simulink model "test_10gbe_mux_pack"  (Simulink 6.2)
settings: Solver=ode45  StartTime=0.0  StopTime=24000  RelTol=1e-3
libraries: xbsIndex_r3 x358, xps_library x31, casper_library x9
(part 1 of 3)
settings Model: LastModifiedBy=manley
settings DebuggingCC: SolverPrmCheckMsg=warning

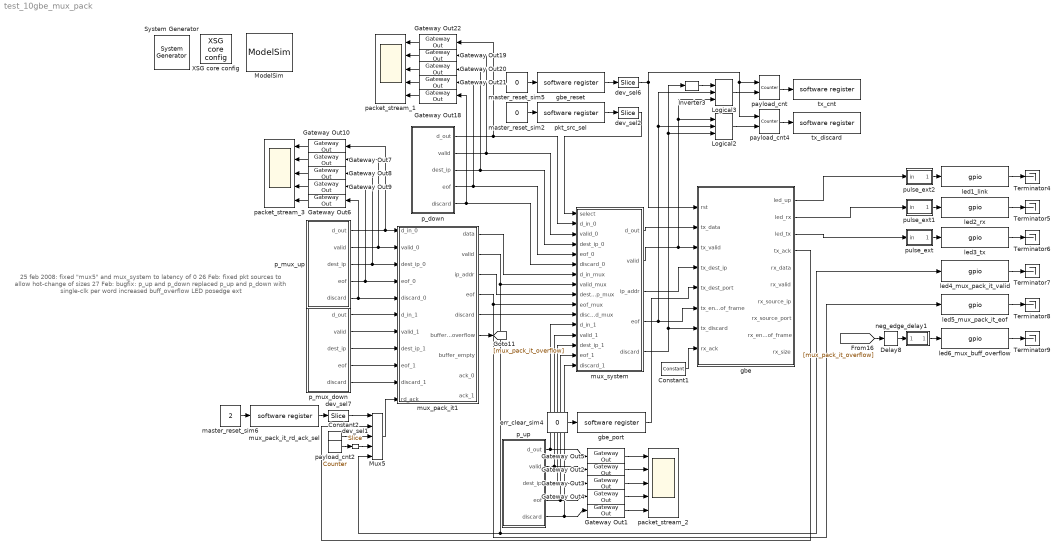
== system test_10gbe_mux_pack ==
  note: 25 feb 2008:
      | fixed "mux5" and mux_system to latency of 0
      |
      | 26 Feb:
      | fixed pkt sources to allow hot-change of sizes
      |
      | 27 Feb:
      | bugfix: p_up and p_down
      | replaced p_up and p_down with single-clk per word
      | increased buff_overflow LED posedge ext
  " System Generator" : xbsIndex_r3/ System Generator  Tag=genX  xilinxfamily=Virtex2P  part=xc2vp70  speed=-7  package=ff1704  synthesis_tool=XST  directory=./test_10gbe_mux_pack/sysgen  testbench=off  simulink_period=1  sysclk_period=4.878  incr_netlist=off  trim_vbits=Everywhere in SubSystem  dbl_ovrd=According to Block Masks  core_generation=According to Block Masks  run_coregen=off  deprecated_control=off  eval_field=0
      settings: AttributesFormatString=System\nGenerator
  Constant1 : xbsIndex_r3/Constant  const=1  equ=P=C  arith_type=Boolean  n_bits=1  bin_pt=0  opselect=C  inp2=PCIN>>17  opr=+  inp1=P  carry=CIN  iostate=0  explicit_period=on  period=1  dbl_ovrd=off
  Constant2 : xbsIndex_r3/Constant  const=1  equ=P=C  arith_type=Boolean  n_bits=1  bin_pt=0  opselect=C  inp2=PCIN>>17  opr=+  inp1=P  carry=CIN  iostate=0  explicit_period=on  period=1  dbl_ovrd=off
  Delay8 : xbsIndex_r3/Delay  latency=1  reg_retiming=off  explicit_period=off  period=1  en=off  accept_only_valid=off  init_zero=on  dbl_ovrd=off  show_param=off
      settings: xl_area=[0, 0, 0, 0, 0, 0, 0]
  Gateway Out{1..5} (5 alike) : xbsIndex_r3/Gateway Out  output_type=Double  nbits=8  bin_pt=6  arith_type=Boolean  quantization=Truncate  overflow=Wrap  hdl_port=on  timing_constraint=None  locs_specified=off  LOCs={}  needs_fixed_name=off  show_param=off
      settings: xl_area=[0, 0, 0, 0, 0, 0, 0]
  Gateway Out{6..10,18..22} (10 alike) : xbsIndex_r3/Gateway Out  Orientation=left  output_type=Double  nbits=8  bin_pt=6  arith_type=Boolean  quantization=Truncate  overflow=Wrap  hdl_port=on  timing_constraint=None  locs_specified=off  LOCs={}  needs_fixed_name=off  show_param=off
      settings: xl_area=[0, 0, 0, 0, 0, 0, 0]
  Inverter3 : xbsIndex_r3/Inverter  latency=0  explicit_period=off  period=1  en=off  dbl_ovrd=off  show_param=off
      settings: xl_area=[0, 0, 0, 0, 0, 0, 0]
  Logical2 : xbsIndex_r3/Logical  logical_function=AND  inputs=3  precision=Full  arith_type=Unsigned  n_bits=8  bin_pt=2  align_bp=on  latency=0  explicit_period=on  period=1  en=off  dbl_ovrd=off  show_param=off
      settings: xl_area=[0, 0, 0, 0, 0, 0, 0]
  Logical3 : xbsIndex_r3/Logical  logical_function=AND  inputs=3  precision=Full  arith_type=Unsigned  n_bits=8  bin_pt=2  align_bp=on  latency=0  explicit_period=on  period=1  en=off  dbl_ovrd=off  show_param=off
      settings: xl_area=[0, 0, 0, 0, 0, 0, 0]
  ModelSim : xbsIndex_r3/ModelSim  dir=./modelsim  waveform=on  leave_open=on  skip_compile=off  custom_scripts=off  startup_timeout=40
  Mux5 : xbsIndex_r3/Mux  inputs=4  precision=Full  arith_type="Signed  (2's comp)"  n_bits=8  bin_pt=2  quantization=Truncate  overflow=Wrap  latency=0  explicit_period=on  period=1  en=off  dbl_ovrd=off  show_param=off  mux_type=off  use_rpm=off  gen_core=off
      settings: xl_area=[0, 0, 0, 0, 0, 0, 0]
  Terminator{4..9} (6 alike) : Terminator
  XSG core config : xps_library/XSG core config  Tag=xps:xsg  hw_sys=BEE2_usr  ibob_linux=off  clk_src=sys_clk2x  gpio_clk_io_group=iBOB:sma  gpio_clk_bit_index=0  clk_rate=205  sample_period=1  synthesis_tool=XST  mpc_type=powerpc405
  dev_sel1 : xbsIndex_r3/Slice  mode=Lower Bit Location + Width  nbits=1  bit1=0  base1=MSB of Input  bit0=0  base0=LSB of Input  boolean_output=on  explicit_period=off  period=1  dbl_ovrd=off
  dev_sel2 : xbsIndex_r3/Slice  mode=Lower Bit Location + Width  nbits=2  bit1=0  base1=MSB of Input  bit0=0  base0=LSB of Input  boolean_output=off  explicit_period=off  period=1  dbl_ovrd=off
  dev_sel6 : xbsIndex_r3/Slice  mode=Lower Bit Location + Width  nbits=1  bit1=0  base1=MSB of Input  bit0=0  base0=LSB of Input  boolean_output=on  explicit_period=off  period=1  dbl_ovrd=off
  dev_sel7 : xbsIndex_r3/Slice  mode=Lower Bit Location + Width  nbits=2  bit1=0  base1=MSB of Input  bit0=0  base0=LSB of Input  boolean_output=off  explicit_period=off  period=1  dbl_ovrd=off
  err_clear_sim4 : Constant  Value=0
  gbe : Subsystem  Tag=xps:tengbe  AncestorBlock=xps_library/ten_GbE  mask{port=BEE2_usr:2, mac_lite=on, show_param=off, pre_emph=3, swing=800}
      mask prompts: mac_lite "Use light-weight MAC: Warning --> it DOES NOT check any CRC on receive"; show_param "---------------------- Show Implementation Parameters -----------------------------------------------------------------------------------"; pre_emph "Pre-emphasis"; swing "Differential swing"
      mask init:
      | tengbe_mask;
      mask StyleString: popup(iBOB:0|iBOB:1|BEE2_ctrl:0|BEE2_ctrl:1|BEE2_usr:0|BEE2_usr:1|BEE2_usr:2|BEE2_usr:3|CORR:0),checkbox,checkbox,popup(0|1|2|3),popup(400|500|600|700|800)
      mask CallbackString:
      | ||myname=gcb;
      | if strcmp(get_param(myname, 'show_param'), 'on')
      |     set_param(myname, 'MaskVisibilities', {'on','on','on','on', 'on'});
      | else
      |     set_param(myname, 'MaskVisibilities', {'on','on','on','off','off'});
      | end||
  gbe_port : xps_library/software register  Tag=xps:sw_reg  io_dir=From Processor  arith_type=Unsigned  bitwidth=32  bin_pt=0  sample_period=1  gw_name=test_10gbe_mux_pack_gbe_port_user_data_out
  gbe_reset : xps_library/software register  Tag=xps:sw_reg  io_dir=From Processor  arith_type=Unsigned  bitwidth=32  bin_pt=0  sample_period=1  gw_name=test_10gbe_mux_pack_gbe_reset_user_data_out
  led1_link : xps_library/gpio  Tag=xps:gpio  io_group=BEE2_usr:led  io_dir=out  arith_type=Boolean  bitwidth=1  bin_pt=0  bit_index=0  sample_period=1  use_single_ended=off  use_ddr=off  reg_iob=off  reg_clk_phase=0  termination=None
  led2_rx : xps_library/gpio  Tag=xps:gpio  io_group=BEE2_usr:led  io_dir=out  arith_type=Boolean  bitwidth=1  bin_pt=0  bit_index=1  sample_period=1  use_single_ended=off  use_ddr=off  reg_iob=off  reg_clk_phase=0  termination=None
  led3_tx : xps_library/gpio  Tag=xps:gpio  io_group=BEE2_usr:led  io_dir=out  arith_type=Boolean  bitwidth=1  bin_pt=0  bit_index=2  sample_period=1  use_single_ended=off  use_ddr=off  reg_iob=off  reg_clk_phase=0  termination=None
  led4_mux_pack_it_valid : xps_library/gpio  Tag=xps:gpio  io_group=BEE2_usr:led  io_dir=out  arith_type=Boolean  bitwidth=1  bin_pt=0  bit_index=3  sample_period=1  use_single_ended=off  use_ddr=off  reg_iob=off  reg_clk_phase=0  termination=None
  led5_mux_pack_it_eof : xps_library/gpio  Tag=xps:gpio  io_group=BEE2_usr:led  io_dir=out  arith_type=Boolean  bitwidth=1  bin_pt=0  bit_index=4  sample_period=1  use_single_ended=off  use_ddr=off  reg_iob=off  reg_clk_phase=0  termination=None
  led6_mux_buff_overflow : xps_library/gpio  Tag=xps:gpio  io_group=BEE2_usr:led  io_dir=out  arith_type=Boolean  bitwidth=1  bin_pt=0  bit_index=5  sample_period=1  use_single_ended=off  use_ddr=off  reg_iob=off  reg_clk_phase=0  termination=None
  master_reset_sim2 : Constant  Value=0
  master_reset_sim5 : Constant  Value=0
  master_reset_sim6 : Constant  Value=2
  mux_pack_it1 : Subsystem  mask(mux_packets){max_packet_size_0=1500, min_packet_size_0=50, max_packet_size_1=1500, min_packet_size_1=50}
      mask prompts: max_packet_size_0 "Input 0: Maximum single packet size (words)"; min_packet_size_0 "Input 0: Minimum single packet size (words)"; max_packet_size_1 "Input 1: Maximum single packet size (words)"; min_packet_size_1 "Input 1: Minimum single packet size (words)"
      mask help: This block allows you to mux together two data streams to be sent to the 10GbE core
  mux_pack_it_rd_ack_sel : xps_library/software register  Tag=xps:sw_reg  io_dir=From Processor  arith_type=Unsigned  bitwidth=32  bin_pt=0  sample_period=1  gw_name=test_10gbe_mux_pack_mux_pack_it_rd_ack_sel_user_data_out
  mux_system : Subsystem
  neg_edge_delay1 : Subsystem  AncestorBlock=casper_library/Misc/pulse_ext  mask(pulse_ext){pulse_len=2^27}
      mask prompts: pulse_len "Length of Pulse"
      mask help:
      | Extends a boolean signal to be high for the specified number of clocks after
      | the last high input.
      mask init:
      | bits = ceil(log2(pulse_len+1));
      mask Help: eval('xlWeb([getenv(''MLIB_ROOT''), ''\casper_library\doc\pulse_ext_usage.html''])')
  p_down : Subsystem
  p_mux_down : Subsystem
  p_mux_up : Subsystem
  p_up : Subsystem
  packet_stream_1 : Scope  NumInputPorts=5
      settings: YMin=4490~0~3.35544e+008~0~-1  YMax=4600~1~3.35544e+008~1~1
  packet_stream_2 : Scope  NumInputPorts=5
      settings: YMin=600~0~3.35544e+008~0~-1  YMax=710~1~3.35544e+008~1~1
  packet_stream_3 : Scope  NumInputPorts=5
      settings: YMin=800~0~3.18767e+008~0~-1  YMax=910~1~3.52321e+008~1~1  SaveName=ScopeData2
  payload_cnt : xbsIndex_r3/Counter  cnt_type=Free Running  n_bits=32  bin_pt=0  arith_type=Unsigned  start_count=0  cnt_to=0  cnt_by_val=1  operation=Up  explicit_period=off  period=1  load_pin=off  rst=on  en=on  dbl_ovrd=off  show_param=off  use_rpm=on  gen_core=off
      settings: xl_area=[0, 0, 0, 0, 0, 0, 0]
  payload_cnt2 : xbsIndex_r3/Counter  cnt_type=Free Running  n_bits=2  bin_pt=0  arith_type=Unsigned  start_count=0  cnt_to=0  cnt_by_val=1  operation=Up  explicit_period=off  period=1  load_pin=off  rst=off  en=off  dbl_ovrd=off  show_param=off  use_rpm=on  gen_core=off
      settings: xl_area=[0, 0, 0, 0, 0, 0, 0]
  payload_cnt4 : xbsIndex_r3/Counter  cnt_type=Free Running  n_bits=32  bin_pt=0  arith_type=Unsigned  start_count=0  cnt_to=0  cnt_by_val=1  operation=Up  explicit_period=off  period=1  load_pin=off  rst=on  en=on  dbl_ovrd=off  show_param=off  use_rpm=on  gen_core=off
      settings: xl_area=[0, 0, 0, 0, 0, 0, 0]
  pkt_src_sel : xps_library/software register  Tag=xps:sw_reg  io_dir=From Processor  arith_type=Unsigned  bitwidth=32  bin_pt=0  sample_period=1  gw_name=test_10gbe_mux_pack_pkt_src_sel_user_data_out
  pulse_ext : Subsystem  mask{pulse_len=2^23}
      mask prompts: pulse_len "Length of Pulse"
      mask init:
      | bits = ceil(log2(pulse_len));
  pulse_ext1 : Subsystem  mask{pulse_len=2^23}
      mask prompts: pulse_len "Length of Pulse"
      mask init:
      | bits = ceil(log2(pulse_len));
  pulse_ext2 : Subsystem  mask{pulse_len=2^23}
      mask prompts: pulse_len "Length of Pulse"
      mask init:
      | bits = ceil(log2(pulse_len));
  tx_cnt : xps_library/software register  Tag=xps:sw_reg  io_dir=To Processor  arith_type=Unsigned  bitwidth=32  bin_pt=0  sample_period=1  gw_name=test_10gbe_mux_pack_tx_cnt_user_data_in
  tx_discard : xps_library/software register  Tag=xps:sw_reg  io_dir=To Processor  arith_type=Unsigned  bitwidth=32  bin_pt=0  sample_period=1  gw_name=test_10gbe_mux_pack_tx_discard_user_data_in
  wires:
  p_down/1(d_out) -> Gateway Out22/1, mux_system/2(d_in_0)
  p_down/2(valid) -> Gateway Out19/1, mux_system/3(valid_0)
  p_down/3(dest_ip) -> Gateway Out20/1, mux_system/4(dest_ip_0)
  p_down/4(eof) -> Gateway Out21/1, mux_system/5(eof_0)
  p_down/5(discard) -> Gateway Out18/1, mux_system/6(discard_0)
  p_up/1(d_out) -> Gateway Out5/1, mux_system/12(d_in_1)
  p_up/2(valid) -> Gateway Out2/1, mux_system/13(valid_1)
  p_up/3(dest_ip) -> Gateway Out3/1, mux_system/14(dest_ip_1)
  p_up/4(eof) -> Gateway Out4/1, mux_system/15(eof_1)
  p_up/5(discard) -> Gateway Out1/1, mux_system/16(discard_1)
  dev_sel6/1 -> gbe/1(rst), payload_cnt/1, payload_cnt4/1
  mux_system/1(d_out) -> gbe/2(tx_data)
  mux_system/2(valid) -> gbe/3(tx_valid), Logical2/1, Logical3/3
  mux_pack_it1/6(buffer_overflow) -> [mux_pack_it_overflow]
  mux_system/3(ip_addr) -> gbe/4(tx_dest_ip)
  mux_system/4(eof) -> Logical2/2, Logical3/2, gbe/6(tx_end_of_frame)
  mux_system/5(discard) -> Inverter3/1, Logical2/3, gbe/7(tx_discard)
  mux_pack_it1/1(data) -> mux_system/7(d_in_mux)
  mux_pack_it1/2(valid) -> Mux5/5, led4_mux_pack_it_valid/1, mux_system/8(valid_mux)
  mux_pack_it1/3(ip_addr) -> mux_system/9(dest_ip_mux)
  mux_pack_it1/4(eof) -> led5_mux_pack_it_eof/1, mux_system/10(eof_mux)
  mux_pack_it1/5(discard) -> mux_system/11(discard_mux)
  Inverter3/1 -> Logical3/1
  payload_cnt/1 -> tx_cnt/1
  payload_cnt4/1 -> tx_discard/1
  Logical2/1 -> payload_cnt4/2
  Logical3/1 -> payload_cnt/2
  master_reset_sim2/1 -> pkt_src_sel/1
  pkt_src_sel/1 -> dev_sel2/1
  master_reset_sim5/1 -> gbe_reset/1
  gbe_reset/1 -> dev_sel6/1
  pulse_ext/1(out) -> led3_tx/1
  pulse_ext1/1(out) -> led2_rx/1
  pulse_ext2/1(out) -> led1_link/1
  led1_link/1 -> Terminator4/1
  led2_rx/1 -> Terminator5/1
  led3_tx/1 -> Terminator6/1
  led4_mux_pack_it_valid/1 -> Terminator7/1
  led5_mux_pack_it_eof/1 -> Terminator8/1
  led6_mux_buff_overflow/1 -> Terminator9/1
  Delay8/1 -> neg_edge_delay1/1(in)
  neg_edge_delay1/1(out) -> led6_mux_buff_overflow/1
  gbe/1(led_up) -> pulse_ext2/1(in)
  gbe/2(led_rx) -> pulse_ext1/1(in)
  gbe/3(led_tx) -> pulse_ext/1(in)
  Constant1/1 -> gbe/8(rx_ack)
  err_clear_sim4/1 -> gbe_port/1
  gbe_port/1 -> gbe/5(tx_dest_port)
  [mux_pack_it_overflow] -> Delay8/1
  master_reset_sim6/1 -> mux_pack_it_rd_ack_sel/1
  mux_pack_it_rd_ack_sel/1 -> dev_sel7/1
  dev_sel7/1 -> Mux5/1
  Constant2/1 -> Mux5/3
  Mux5/1 -> mux_pack_it1/11(rd_ack)
  dev_sel2/1 -> mux_system/1(select)
  Gateway Out22/1 -> packet_stream_1/1
  Gateway Out19/1 -> packet_stream_1/2
  Gateway Out20/1 -> packet_stream_1/3
  Gateway Out21/1 -> packet_stream_1/4
  Gateway Out18/1 -> packet_stream_1/5
  Gateway Out5/1 -> packet_stream_2/1
  Gateway Out2/1 -> packet_stream_2/2
  Gateway Out3/1 -> packet_stream_2/3
  Gateway Out4/1 -> packet_stream_2/4
  Gateway Out1/1 -> packet_stream_2/5
  gbe/4(tx_ack) -> Mux5/2
  payload_cnt2/1 -> dev_sel1/1
  dev_sel1/1 -> Mux5/4
  p_mux_up/1(d_out) -> mux_pack_it1/1(d_in_0), Gateway Out10/1
  p_mux_up/2(valid) -> mux_pack_it1/2(valid_0), Gateway Out7/1
  p_mux_up/3(dest_ip) -> mux_pack_it1/3(dest_ip_0), Gateway Out8/1
  p_mux_up/4(eof) -> mux_pack_it1/4(eof_0), Gateway Out9/1
  p_mux_up/5(discard) -> mux_pack_it1/5(discard_0), Gateway Out6/1
  p_mux_down/1(d_out) -> mux_pack_it1/6(d_in_1)
  p_mux_down/2(valid) -> mux_pack_it1/7(valid_1)
  p_mux_down/3(dest_ip) -> mux_pack_it1/8(dest_ip_1)
  p_mux_down/4(eof) -> mux_pack_it1/9(eof_1)
  p_mux_down/5(discard) -> mux_pack_it1/10(discard_1)
  Gateway Out10/1 -> packet_stream_3/1
  Gateway Out7/1 -> packet_stream_3/2
  Gateway Out8/1 -> packet_stream_3/3
  Gateway Out9/1 -> packet_stream_3/4
  Gateway Out6/1 -> packet_stream_3/5

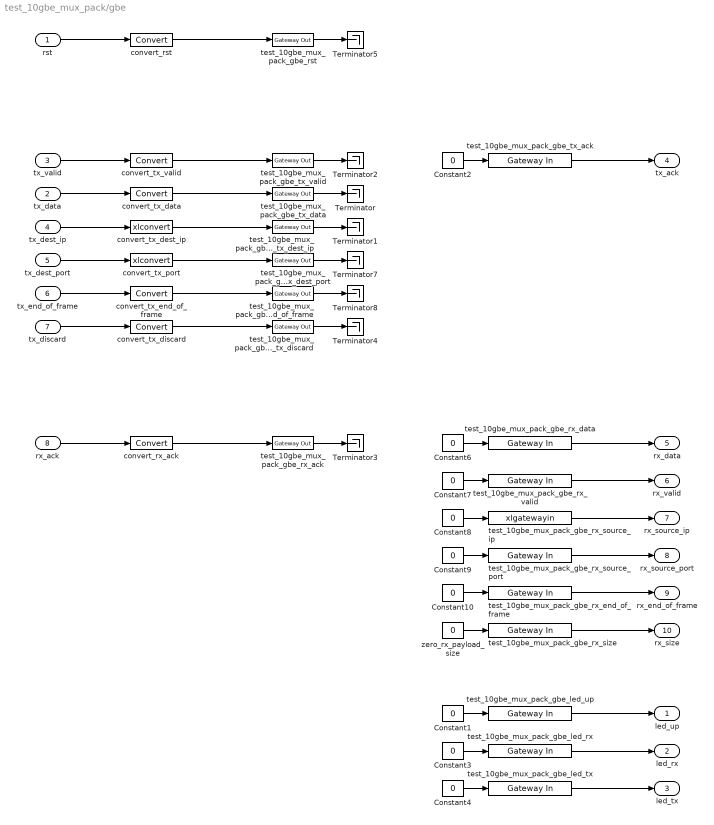
== system test_10gbe_mux_pack/gbe ==
  rst : Inport  Port=1  LatchInput=off
  tx_data : Inport  Port=2  LatchInput=off
  tx_valid : Inport  Port=3  LatchInput=off
  tx_dest_ip : Inport  Port=4  LatchInput=off
  tx_dest_port : Inport  Port=5  LatchInput=off
  tx_end_of_frame : Inport  Port=6  LatchInput=off
  tx_discard : Inport  Port=7  LatchInput=off
  rx_ack : Inport  Port=8  LatchInput=off
  Constant{1..4,6..10} (9 alike) : Constant  Value=0
  Terminator{,1..5,7..8} (8 alike) : Terminator
  convert_rst : xbsIndex_r3/Convert  arith_type=Boolean  n_bits=64  bin_pt=0  quantization=Truncate  overflow=Wrap  latency=0  explicit_period=off  period=1  dbl_ovrd=off  show_param=off  inserted_by_tool=off  pipeline=off
      settings: xl_area=[0, 0, 0, 0, 0, 0, 0]
  convert_rx_ack : xbsIndex_r3/Convert  arith_type=Boolean  n_bits=64  bin_pt=0  quantization=Truncate  overflow=Wrap  latency=0  explicit_period=off  period=1  dbl_ovrd=off  show_param=off  inserted_by_tool=off  pipeline=off
      settings: xl_area=[0, 0, 0, 0, 0, 0, 0]
  convert_tx_data : xbsIndex_r3/Convert  arith_type=Unsigned  n_bits=64  bin_pt=0  quantization=Truncate  overflow=Wrap  latency=0  explicit_period=off  period=1  dbl_ovrd=off  show_param=off  inserted_by_tool=off  pipeline=off
      settings: xl_area=[0, 0, 0, 0, 0, 0, 0]
  convert_tx_dest_ip : S-Function  AncestorBlock=xbsIndex_r3/Convert  FunctionName=xlconvert  Parameters=sfcn_mwsv__  mask(Xilinx Converter Block){arith_type=Unsigned, n_bits=32, bin_pt=0, quantization=Truncate, overflow=Wrap, latency=0, explicit_period=off, period=1, dbl_ovrd=off, show_param=off, inserted_by_tool=off, pipeline=off, xl_area=[0, 0, 0, 0, 0, 0, 0], xl_use_area=off}
      mask prompts: arith_type "Output Type"; n_bits "Number of Bits"; bin_pt "Binary Point"; quantization "Quantization Behavior"; overflow "Overflow Behavior"; explicit_period "Use Explicit Sample Period"; period "Sample Period"; dbl_ovrd "Override with Doubles"; show_param "---------------------- Show Implementation Parameters -----------------------------------------------------------------------------------"; inserted_by_tool "Hidden Parameter:  inserted_by_tool"; pipeline "Pipeline to Greatest Extent Possible"; xl_area "FPGA Area [Slices, FFs, BRAMs, LUTs, IOBs, Emb. Mults, TBUFs]"; xl_use_area "Use Area Above For Estimation"
      mask help:
      | Type conversion block. The input is presented at the output after quantization and overflow effects.
      |
      | Hardware notes: Additional hardware is used when rounding or saturation is selected and output width is less than the input width.
      mask init:
      | [designRoot, family, part, speed, package, simulinkPeriod, sysclkPeriod, dbl_ovrd, trimVbit] = xlSysgenSettings(gcb,1,1);
      | if (arith_type==1)
      |   bool = 1;
      | else
      |   bool = 0;
      |   arith_type = arith_type-1;
      | end
      | zstr=''; zpstr='';
      | if latency > 0
      |   zstr = 'z';
      |   zpstr = sprintf('-%d', latency);
      | end
      | [bg,fg] = xlcmap('XBlock',dbl_ovrd);
      | if (inserted_by_tool)
      |   bg = [1.00 0.50 0.25];
      | end
      | iPos = get_param(gcb,'Position');
      | iWidth=iPos(3)-iPos(1); iHeight=iPos(4)-iPos(2);
      | iCx=iWidth/2;
      | iCy=iHeight/2;
      | [logoX, logoY] = xlogo(iPos);
      | zstrx = 0.45*iWidth-11; if (zstrx<3) zstrx=3; end
      | zstry = 0.36*iHeight-7; if (zstry<3) zstry=3; end
      | 
      | 
      | % one time added for param list
      | dblOvrd = dbl_ovrd;
      | precision0 = 2;
      | z0 = [n_bits bin_pt arith_type quantization overflow];
      | explicitClk = explicit_period;
      | 
      | 
      | % just pass everything to s-function
      | sfcn_mwsv__ = get_param(gcb, 'MaskWSVariables');
      mask Help: eval('xlWeb(xlhtmldoclink(''Convert''))');
      mask StyleString: popup(Boolean|Unsigned|Signed  (2's comp)),edit,edit,popup(Truncate|Round  (unbiased: +/- Inf)|Round  (unbiased: Even Values)),popup(Wrap|Saturate|Error),edit,checkbox,edit,checkbox,checkbox,checkbox,checkbox,edit,checkbox
      mask CallbackString: xlconvertCallback||||||xlMagicCallback|||xlShowIPCallback||||
      mask Display:
      | patch([0 iWidth iWidth 0],[0 0 iHeight iHeight] , bg);
      | patch(logoX,logoY , fg);
      | text(zstrx,zstry,zstr);
      | text(zstrx+5,zstry+5,zpstr);
      | port_label('output',1,'cast');
      | plot([0 0 iWidth iWidth 0], [0 iHeight iHeight 0 0]);
  convert_tx_discard : xbsIndex_r3/Convert  arith_type=Boolean  n_bits=1  bin_pt=0  quantization=Truncate  overflow=Wrap  latency=0  explicit_period=off  period=1  dbl_ovrd=off  show_param=off  inserted_by_tool=off  pipeline=off
      settings: xl_area=[0, 0, 0, 0, 0, 0, 0]
  convert_tx_end_of_frame : xbsIndex_r3/Convert  arith_type=Boolean  n_bits=1  bin_pt=0  quantization=Truncate  overflow=Wrap  latency=0  explicit_period=off  period=1  dbl_ovrd=off  show_param=off  inserted_by_tool=off  pipeline=off
      settings: xl_area=[0, 0, 0, 0, 0, 0, 0]
  convert_tx_port : S-Function  AncestorBlock=xbsIndex_r3/Convert  FunctionName=xlconvert  Parameters=sfcn_mwsv__  mask(Xilinx Converter Block){arith_type=Unsigned, n_bits=16, bin_pt=0, quantization=Truncate, overflow=Wrap, latency=0, explicit_period=off, period=1, dbl_ovrd=off, show_param=off, inserted_by_tool=off, pipeline=off, xl_area=[0, 0, 0, 0, 0, 0, 0], xl_use_area=off}
      mask prompts: arith_type "Output Type"; n_bits "Number of Bits"; bin_pt "Binary Point"; quantization "Quantization Behavior"; overflow "Overflow Behavior"; explicit_period "Use Explicit Sample Period"; period "Sample Period"; dbl_ovrd "Override with Doubles"; show_param "---------------------- Show Implementation Parameters -----------------------------------------------------------------------------------"; inserted_by_tool "Hidden Parameter:  inserted_by_tool"; pipeline "Pipeline to Greatest Extent Possible"; xl_area "FPGA Area [Slices, FFs, BRAMs, LUTs, IOBs, Emb. Mults, TBUFs]"; xl_use_area "Use Area Above For Estimation"
      mask help:
      | Type conversion block. The input is presented at the output after quantization and overflow effects.
      |
      | Hardware notes: Additional hardware is used when rounding or saturation is selected and output width is less than the input width.
      mask init: same as test_10gbe_mux_pack/gbe/convert_tx_dest_ip
      mask Help: eval('xlWeb(xlhtmldoclink(''Convert''))');
      mask StyleString: popup(Boolean|Unsigned|Signed  (2's comp)),edit,edit,popup(Truncate|Round  (unbiased: +/- Inf)|Round  (unbiased: Even Values)),popup(Wrap|Saturate|Error),edit,checkbox,edit,checkbox,checkbox,checkbox,checkbox,edit,checkbox
      mask CallbackString: xlconvertCallback||||||xlMagicCallback|||xlShowIPCallback||||
      mask Display:
      | patch([0 iWidth iWidth 0],[0 0 iHeight iHeight] , bg);
      | patch(logoX,logoY , fg);
      | text(zstrx,zstry,zstr);
      | text(zstrx+5,zstry+5,zpstr);
      | port_label('output',1,'cast');
      | plot([0 0 iWidth iWidth 0], [0 iHeight iHeight 0 0]);
  convert_tx_valid : xbsIndex_r3/Convert  arith_type=Boolean  n_bits=1  bin_pt=0  quantization=Truncate  overflow=Wrap  latency=0  explicit_period=off  period=1  dbl_ovrd=off  show_param=off  inserted_by_tool=off  pipeline=off
      settings: xl_area=[0, 0, 0, 0, 0, 0, 0]
  test_10gbe_mux_pack_gbe_led_rx : xbsIndex_r3/Gateway In  arith_type=Boolean  n_bits=1  bin_pt=0  quantization=Truncate  overflow=Wrap  period=1  timing_constraint=None  locs_specified=off  LOCs={}  needs_fixed_name=off  dbl_ovrd=off  show_param=off
      settings: xl_area=[0, 0, 0, 0, 0, 0, 0]
  test_10gbe_mux_pack_gbe_led_tx : xbsIndex_r3/Gateway In  arith_type=Boolean  n_bits=1  bin_pt=0  quantization=Truncate  overflow=Wrap  period=1  timing_constraint=None  locs_specified=off  LOCs={}  needs_fixed_name=off  dbl_ovrd=off  show_param=off
      settings: xl_area=[0, 0, 0, 0, 0, 0, 0]
  test_10gbe_mux_pack_gbe_led_up : xbsIndex_r3/Gateway In  arith_type=Boolean  n_bits=1  bin_pt=0  quantization=Truncate  overflow=Wrap  period=1  timing_constraint=None  locs_specified=off  LOCs={}  needs_fixed_name=off  dbl_ovrd=off  show_param=off
      settings: xl_area=[0, 0, 0, 0, 0, 0, 0]
  test_10gbe_mux_pack_gbe_rst : xbsIndex_r3/Gateway Out  output_type=Double  nbits=8  bin_pt=6  arith_type=Boolean  quantization=Truncate  overflow=Wrap  hdl_port=on  timing_constraint=None  locs_specified=off  LOCs={}  needs_fixed_name=off  show_param=off
      settings: xl_area=[0, 0, 0, 0, 0, 0, 0]
  test_10gbe_mux_pack_gbe_rx_ack : xbsIndex_r3/Gateway Out  output_type=Double  nbits=8  bin_pt=6  arith_type=Boolean  quantization=Truncate  overflow=Wrap  hdl_port=on  timing_constraint=None  locs_specified=off  LOCs={}  needs_fixed_name=off  show_param=off
      settings: xl_area=[0, 0, 0, 0, 0, 0, 0]
  test_10gbe_mux_pack_gbe_rx_data : xbsIndex_r3/Gateway In  arith_type=Unsigned  n_bits=64  bin_pt=0  quantization=Truncate  overflow=Wrap  period=1  timing_constraint=None  locs_specified=off  LOCs={}  needs_fixed_name=off  dbl_ovrd=off  show_param=off
      settings: xl_area=[0, 0, 0, 0, 0, 0, 0]
  test_10gbe_mux_pack_gbe_rx_end_of_frame : xbsIndex_r3/Gateway In  arith_type=Boolean  n_bits=1  bin_pt=0  quantization=Truncate  overflow=Wrap  period=1  timing_constraint=None  locs_specified=off  LOCs={}  needs_fixed_name=off  dbl_ovrd=off  show_param=off
      settings: xl_area=[0, 0, 0, 0, 0, 0, 0]
  test_10gbe_mux_pack_gbe_rx_size : xbsIndex_r3/Gateway In  arith_type=Unsigned  n_bits=16  bin_pt=0  quantization=Truncate  overflow=Wrap  period=1  timing_constraint=None  locs_specified=off  LOCs={}  needs_fixed_name=off  dbl_ovrd=off  show_param=off
      settings: xl_area=[0, 0, 0, 0, 0, 0, 0]
  test_10gbe_mux_pack_gbe_rx_source_ip : S-Function  AncestorBlock=xbsIndex_r3/Gateway In  FunctionName=xlgatewayin  Parameters="arith_type, n_bits, bin_pt, quantization, overflow,  gcb, period, dbl_ovrd, locs_specified, LOCs, timing_constraint, simulinkPeriod, designRoot, 0"  mask(Xilinx Gateway In){arith_type=Unsigned, n_bits=32, bin_pt=0, quantization=Truncate, overflow=Wrap, period=1, timing_constraint=None, locs_specified=off, LOCs={}, needs_fixed_name=off, dbl_ovrd=off, show_param=off, xl_area=[0, 0, 0, 0, 0, 0, 0], xl_use_area=off}
      mask prompts: arith_type "Output Data Type"; n_bits "Number of Bits"; bin_pt "Binary Point"; period "Sample Period"; timing_constraint "IOB Timing Constraint"; locs_specified "Specify IOB Location Constraints"; LOCs "IOB Pad Locations (specify as cell array {'MSB', ..., 'LSB'})"; needs_fixed_name "Do Not Prepend Hierarchy to Port Name"; dbl_ovrd "Override with Double"; show_param "---------------------- Show Implementation Parameters -----------------------------------------------------------------------------------"; xl_area "FPGA Area [Slices, FFs, BRAMs, LUTs, IOBs, Emb. Mults, TBUFs]"; xl_use_area "Use Area Above For Estimation"
      mask help:
      | Gateway in block.  Converts inputs of type Simulink integer, double and fixed point to  Xilinx fixed point type.
      |
      | Hardware notes:  In hardware these blocks become top level input ports.
      mask init:
      | [designRoot, family, part, speed, package, simulinkPeriod, sysclkPeriod, dbl_ovrd, trimVbit] = xlSysgenSettings(gcb,1,0);
      | trimVbit = 1;
      | [bg,fg] = xlcmap('IO',dbl_ovrd);
      | iPos = get_param(gcb,'Position');
      | iWidth=iPos(3)-iPos(1); iHeight=iPos(4)-iPos(2);
      | iCx=iWidth/2;
      | iCy=iHeight/2;
      | [logoX, logoY] = xlogo(iPos);
      mask Help: eval('xlWeb(xlhtmldoclink(''Gateway In''))');
      mask StyleString: popup(Boolean|Unsigned|Signed  (2's comp)),edit,edit,popup(Truncate|Round  (unbiased: +/- Inf)),popup(Wrap|Saturate|Flag as Error),edit,popup(None|Data Rate|Data Rate;  Set 'FAST' Attribute),checkbox,edit,checkbox,checkbox,checkbox,edit,checkbox
      mask CallbackString: xlgatewayinCallback|||||||xlgatewayinCallback||||xlShowIPCallback||
      mask Display:
      | patch([0 iWidth iWidth 0],[0 0 iHeight iHeight] , bg);
      | patch(logoX,logoY , fg);
      | port_label('input',1,'dbl');
      | port_label('output',1,'fpt');
      | 
      | ;plot([0 0 iWidth iWidth 0], [0 iHeight iHeight 0 0]);
  test_10gbe_mux_pack_gbe_rx_source_port : xbsIndex_r3/Gateway In  arith_type=Unsigned  n_bits=16  bin_pt=0  quantization=Truncate  overflow=Wrap  period=1  timing_constraint=None  locs_specified=off  LOCs={}  needs_fixed_name=off  dbl_ovrd=off  show_param=off
      settings: xl_area=[0, 0, 0, 0, 0, 0, 0]
  test_10gbe_mux_pack_gbe_rx_valid : xbsIndex_r3/Gateway In  arith_type=Boolean  n_bits=1  bin_pt=0  quantization=Truncate  overflow=Wrap  period=1  timing_constraint=None  locs_specified=off  LOCs={}  needs_fixed_name=off  dbl_ovrd=off  show_param=off
      settings: xl_area=[0, 0, 0, 0, 0, 0, 0]
  test_10gbe_mux_pack_gbe_tx_ack : xbsIndex_r3/Gateway In  arith_type=Boolean  n_bits=1  bin_pt=0  quantization=Truncate  overflow=Wrap  period=1  timing_constraint=None  locs_specified=off  LOCs={}  needs_fixed_name=off  dbl_ovrd=off  show_param=off
      settings: xl_area=[0, 0, 0, 0, 0, 0, 0]
  test_10gbe_mux_pack_gbe_tx_data : xbsIndex_r3/Gateway Out  output_type=Double  nbits=8  bin_pt=6  arith_type=Boolean  quantization=Truncate  overflow=Wrap  hdl_port=on  timing_constraint=None  locs_specified=off  LOCs={}  needs_fixed_name=off  show_param=off
      settings: xl_area=[0, 0, 0, 0, 0, 0, 0]
  test_10gbe_mux_pack_gbe_tx_dest_ip : xbsIndex_r3/Gateway Out  output_type=Double  nbits=8  bin_pt=6  arith_type=Boolean  quantization=Truncate  overflow=Wrap  hdl_port=on  timing_constraint=None  locs_specified=off  LOCs={}  needs_fixed_name=off  show_param=off
      settings: xl_area=[0, 0, 0, 0, 0, 0, 0]
  test_10gbe_mux_pack_gbe_tx_dest_port : xbsIndex_r3/Gateway Out  output_type=Double  nbits=8  bin_pt=6  arith_type=Boolean  quantization=Truncate  overflow=Wrap  hdl_port=on  timing_constraint=None  locs_specified=off  LOCs={}  needs_fixed_name=off  show_param=off
      settings: xl_area=[0, 0, 0, 0, 0, 0, 0]
  test_10gbe_mux_pack_gbe_tx_discard : xbsIndex_r3/Gateway Out  output_type=Double  nbits=8  bin_pt=6  arith_type=Boolean  quantization=Truncate  overflow=Wrap  hdl_port=on  timing_constraint=None  locs_specified=off  LOCs={}  needs_fixed_name=off  show_param=off
      settings: xl_area=[0, 0, 0, 0, 0, 0, 0]
  test_10gbe_mux_pack_gbe_tx_end_of_frame : xbsIndex_r3/Gateway Out  output_type=Double  nbits=8  bin_pt=6  arith_type=Boolean  quantization=Truncate  overflow=Wrap  hdl_port=on  timing_constraint=None  locs_specified=off  LOCs={}  needs_fixed_name=off  show_param=off
      settings: xl_area=[0, 0, 0, 0, 0, 0, 0]
  test_10gbe_mux_pack_gbe_tx_valid : xbsIndex_r3/Gateway Out  output_type=Double  nbits=8  bin_pt=6  arith_type=Boolean  quantization=Truncate  overflow=Wrap  hdl_port=on  timing_constraint=None  locs_specified=off  LOCs={}  needs_fixed_name=off  show_param=off
      settings: xl_area=[0, 0, 0, 0, 0, 0, 0]
  zero_rx_payload_size : Constant  Value=0
  led_up : Outport
  led_rx : Outport  Port=2
  led_tx : Outport  Port=3
  tx_ack : Outport  Port=4
  rx_data : Outport  Port=5
  rx_valid : Outport  Port=6
  rx_source_ip : Outport  Port=7
  rx_source_port : Outport  Port=8
  rx_end_of_frame : Outport  Port=9
  rx_size : Outport  Port=10
  wires:
  test_10gbe_mux_pack_gbe_tx_discard/1 -> Terminator4/1
  convert_tx_discard/1 -> test_10gbe_mux_pack_gbe_tx_discard/1
  tx_discard/1 -> convert_tx_discard/1
  test_10gbe_mux_pack_gbe_rx_size/1 -> rx_size/1
  zero_rx_payload_size/1 -> test_10gbe_mux_pack_gbe_rx_size/1
  test_10gbe_mux_pack_gbe_led_tx/1 -> led_tx/1
  Constant4/1 -> test_10gbe_mux_pack_gbe_led_tx/1
  test_10gbe_mux_pack_gbe_led_rx/1 -> led_rx/1
  Constant3/1 -> test_10gbe_mux_pack_gbe_led_rx/1
  test_10gbe_mux_pack_gbe_led_up/1 -> led_up/1
  Constant1/1 -> test_10gbe_mux_pack_gbe_led_up/1
  test_10gbe_mux_pack_gbe_rx_end_of_frame/1 -> rx_end_of_frame/1
  Constant10/1 -> test_10gbe_mux_pack_gbe_rx_end_of_frame/1
  test_10gbe_mux_pack_gbe_rx_source_port/1 -> rx_source_port/1
  Constant9/1 -> test_10gbe_mux_pack_gbe_rx_source_port/1
  Constant8/1 -> test_10gbe_mux_pack_gbe_rx_source_ip/1
  test_10gbe_mux_pack_gbe_rx_source_ip/1 -> rx_source_ip/1
  test_10gbe_mux_pack_gbe_tx_end_of_frame/1 -> Terminator8/1
  convert_tx_end_of_frame/1 -> test_10gbe_mux_pack_gbe_tx_end_of_frame/1
  tx_end_of_frame/1 -> convert_tx_end_of_frame/1
  test_10gbe_mux_pack_gbe_tx_dest_port/1 -> Terminator7/1
  convert_tx_port/1 -> test_10gbe_mux_pack_gbe_tx_dest_port/1
  tx_dest_port/1 -> convert_tx_port/1
  test_10gbe_mux_pack_gbe_rst/1 -> Terminator5/1
  convert_rst/1 -> test_10gbe_mux_pack_gbe_rst/1
  rst/1 -> convert_rst/1
  test_10gbe_mux_pack_gbe_rx_valid/1 -> rx_valid/1
  Constant7/1 -> test_10gbe_mux_pack_gbe_rx_valid/1
  test_10gbe_mux_pack_gbe_rx_ack/1 -> Terminator3/1
  Constant6/1 -> test_10gbe_mux_pack_gbe_rx_data/1
  Constant2/1 -> test_10gbe_mux_pack_gbe_tx_ack/1
  test_10gbe_mux_pack_gbe_tx_valid/1 -> Terminator2/1
  test_10gbe_mux_pack_gbe_tx_dest_ip/1 -> Terminator1/1
  test_10gbe_mux_pack_gbe_tx_data/1 -> Terminator/1
  test_10gbe_mux_pack_gbe_tx_ack/1 -> tx_ack/1
  convert_tx_valid/1 -> test_10gbe_mux_pack_gbe_tx_valid/1
  tx_valid/1 -> convert_tx_valid/1
  convert_tx_dest_ip/1 -> test_10gbe_mux_pack_gbe_tx_dest_ip/1
  tx_dest_ip/1 -> convert_tx_dest_ip/1
  convert_tx_data/1 -> test_10gbe_mux_pack_gbe_tx_data/1
  tx_data/1 -> convert_tx_data/1
  test_10gbe_mux_pack_gbe_rx_data/1 -> rx_data/1
  convert_rx_ack/1 -> test_10gbe_mux_pack_gbe_rx_ack/1
  rx_ack/1 -> convert_rx_ack/1

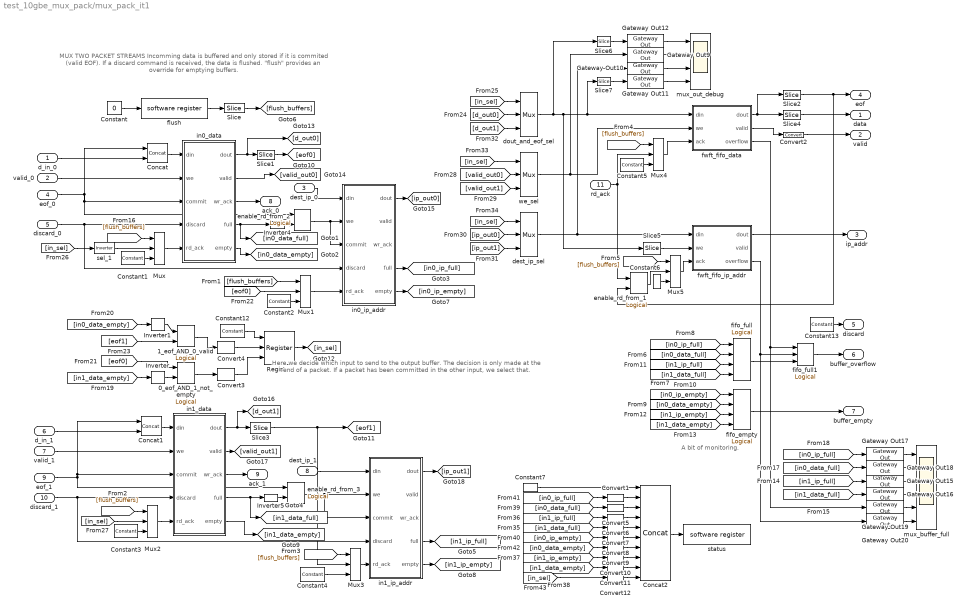
== system test_10gbe_mux_pack/mux_pack_it1 ==
  note: Here we decide which input
      | to send to the output buffer.
      | The decision is only made at the end of a packet.
      | If a packet has been committed in the other input,
      | we select that.
  note: A bit of monitoring.
  note: MUX TWO PACKET STREAMS
      | Incomming data is buffered and only stored if it is commited (valid EOF).
      | If a discard command is received, the data is flushed.
      | "flush" provides an override for emptying buffers.
  d_in_0 : Inport  Port=1  LatchInput=off
  valid_0 : Inport  Port=2  LatchInput=off
  dest_ip_0 : Inport  Port=3  LatchInput=off
  eof_0 : Inport  Port=4  LatchInput=off
  discard_0 : Inport  Port=5  LatchInput=off
  d_in_1 : Inport  Port=6  LatchInput=off
  valid_1 : Inport  Port=7  LatchInput=off
  dest_ip_1 : Inport  Port=8  LatchInput=off
  eof_1 : Inport  Port=9  LatchInput=off
  discard_1 : Inport  Port=10  LatchInput=off
  rd_ack : Inport  Port=11  LatchInput=off
  0_eof_AND_1_not_empty : xbsIndex_r3/Logical  logical_function=AND  inputs=2  precision=Full  arith_type=Unsigned  n_bits=8  bin_pt=2  align_bp=on  latency=0  explicit_period=on  period=1  en=off  dbl_ovrd=off  show_param=off
      settings: xl_area=[0, 0, 0, 0, 0, 0, 0]
  1_eof_AND_0_valid : xbsIndex_r3/Logical  logical_function=AND  inputs=2  precision=Full  arith_type=Unsigned  n_bits=8  bin_pt=2  align_bp=on  latency=0  explicit_period=on  period=1  en=off  dbl_ovrd=off  show_param=off
      settings: xl_area=[0, 0, 0, 0, 0, 0, 0]
  Concat : xbsIndex_r3/Concat  num_inputs=2  explicit_period=off  period=1  dbl_ovrd=off
  Concat1 : xbsIndex_r3/Concat  num_inputs=2  explicit_period=off  period=1  dbl_ovrd=off
  Concat2 : xbsIndex_r3/Concat  num_inputs=10  explicit_period=off  period=1  dbl_ovrd=off
  Constant : Constant  Value=0
  Constant{1..6,12} (7 alike) : xbsIndex_r3/Constant  const=1  equ=P=C  arith_type=Boolean  n_bits=1  bin_pt=0  opselect=C  inp2=PCIN>>17  opr=+  inp1=P  carry=CIN  iostate=0  explicit_period=on  period=1  dbl_ovrd=off
  Constant13 : xbsIndex_r3/Constant  const=0  equ=P=C  arith_type=Boolean  n_bits=1  bin_pt=0  opselect=C  inp2=PCIN>>17  opr=+  inp1=P  carry=CIN  iostate=0  explicit_period=on  period=1  dbl_ovrd=off
  Constant7 : xbsIndex_r3/Constant  const=0  equ=P=C  arith_type=Unsigned  n_bits=32-9  bin_pt=0  opselect=C  inp2=PCIN>>17  opr=+  inp1=P  carry=CIN  iostate=0  explicit_period=on  period=1  dbl_ovrd=off
  Convert{1,5..12} (9 alike) : xbsIndex_r3/Convert  arith_type=Unsigned  n_bits=1  bin_pt=0  quantization=Truncate  overflow=Wrap  latency=0  explicit_period=off  period=1  dbl_ovrd=off  show_param=off  inserted_by_tool=off  pipeline=off
      settings: xl_area=[0, 0, 0, 0, 0, 0, 0]
  Convert2 : xbsIndex_r3/Convert  arith_type=Boolean  n_bits=8  bin_pt=6  quantization=Truncate  overflow=Wrap  latency=0  explicit_period=off  period=1  dbl_ovrd=off  show_param=off  inserted_by_tool=off  pipeline=off
      settings: xl_area=[0, 0, 0, 0, 0, 0, 0]
  Convert3 : xbsIndex_r3/Convert  arith_type=Boolean  n_bits=8  bin_pt=6  quantization=Truncate  overflow=Wrap  latency=0  explicit_period=off  period=1  dbl_ovrd=off  show_param=off  inserted_by_tool=off  pipeline=off
      settings: xl_area=[0, 0, 0, 0, 0, 0, 0]
  Convert4 : xbsIndex_r3/Convert  arith_type=Boolean  n_bits=8  bin_pt=6  quantization=Truncate  overflow=Wrap  latency=0  explicit_period=off  period=1  dbl_ovrd=off  show_param=off  inserted_by_tool=off  pipeline=off
      settings: xl_area=[0, 0, 0, 0, 0, 0, 0]
  Gateway Out{9..12,15..20} (10 alike) : xbsIndex_r3/Gateway Out  output_type=Double  nbits=8  bin_pt=6  arith_type=Boolean  quantization=Truncate  overflow=Wrap  hdl_port=on  timing_constraint=None  locs_specified=off  LOCs={}  needs_fixed_name=off  show_param=off
      settings: xl_area=[0, 0, 0, 0, 0, 0, 0]
  Inverter{,1,4..5} (4 alike) : xbsIndex_r3/Inverter  latency=0  explicit_period=off  period=1  en=off  dbl_ovrd=off  show_param=off
      settings: xl_area=[0, 0, 0, 0, 0, 0, 0]
  Mux{,1..5} (6 alike) : xbsIndex_r3/Mux  inputs=2  precision=Full  arith_type="Signed  (2's comp)"  n_bits=8  bin_pt=2  quantization=Truncate  overflow=Wrap  latency=0  explicit_period=on  period=1  en=off  dbl_ovrd=off  show_param=off  mux_type=off  use_rpm=off  gen_core=off
      settings: xl_area=[0, 0, 0, 0, 0, 0, 0]
  Register : xbsIndex_r3/Register  init=0  reg_only_valid=off  explicit_period=on  period=1  rst=on  en=on  out_en=off  dbl_ovrd=off  show_param=off
      settings: xl_area=[0, 0, 0, 0, 0, 0, 0]
  Slice : xbsIndex_r3/Slice  mode=Lower Bit Location + Width  nbits=1  bit1=0  base1=MSB of Input  bit0=0  base0=LSB of Input  boolean_output=on  explicit_period=off  period=1  dbl_ovrd=off
  Slice{1..3,5} (4 alike) : xbsIndex_r3/Slice  mode=Upper Bit Location + Width  nbits=1  bit1=0  base1=MSB of Input  bit0=0  base0=LSB of Input  boolean_output=on  explicit_period=off  period=1  dbl_ovrd=off
  Slice4 : xbsIndex_r3/Slice  mode=Lower Bit Location + Width  nbits=64  bit1=0  base1=MSB of Input  bit0=0  base0=LSB of Input  boolean_output=off  explicit_period=off  period=1  dbl_ovrd=off
  Slice6 : xbsIndex_r3/Slice  mode=Lower Bit Location + Width  nbits=64  bit1=0  base1=MSB of Input  bit0=0  base0=LSB of Input  boolean_output=off  explicit_period=off  period=1  dbl_ovrd=off
  Slice7 : xbsIndex_r3/Slice  mode=Upper Bit Location + Width  nbits=1  bit1=0  base1=MSB of Input  bit0=0  base0=LSB of Input  boolean_output=off  explicit_period=off  period=1  dbl_ovrd=off
  dest_ip_sel : xbsIndex_r3/Mux  inputs=2  precision=Full  arith_type="Signed  (2's comp)"  n_bits=8  bin_pt=2  quantization=Truncate  overflow=Wrap  latency=0  explicit_period=off  period=1  en=off  dbl_ovrd=off  show_param=off  mux_type=off  use_rpm=off  gen_core=off
      settings: xl_area=[0, 0, 0, 0, 0, 0, 0]
  dout_and_eof_sel : xbsIndex_r3/Mux  inputs=2  precision=Full  arith_type="Signed  (2's comp)"  n_bits=8  bin_pt=2  quantization=Truncate  overflow=Wrap  latency=0  explicit_period=off  period=1  en=off  dbl_ovrd=off  show_param=off  mux_type=off  use_rpm=off  gen_core=off
      settings: xl_area=[0, 0, 0, 0, 0, 0, 0]
  enable_rd_from_1 : xbsIndex_r3/Logical  logical_function=AND  inputs=2  precision=Full  arith_type=Unsigned  n_bits=8  bin_pt=2  align_bp=on  latency=0  explicit_period=off  period=1  en=off  dbl_ovrd=off  show_param=off
      settings: xl_area=[0, 0, 0, 0, 0, 0, 0]
  enable_rd_from_2 : xbsIndex_r3/Logical  logical_function=AND  inputs=2  precision=Full  arith_type=Unsigned  n_bits=8  bin_pt=2  align_bp=on  latency=0  explicit_period=off  period=1  en=off  dbl_ovrd=off  show_param=off
      settings: xl_area=[0, 0, 0, 0, 0, 0, 0]
  enable_rd_from_3 : xbsIndex_r3/Logical  logical_function=AND  inputs=2  precision=Full  arith_type=Unsigned  n_bits=8  bin_pt=2  align_bp=on  latency=0  explicit_period=off  period=1  en=off  dbl_ovrd=off  show_param=off
      settings: xl_area=[0, 0, 0, 0, 0, 0, 0]
  fifo_empty : xbsIndex_r3/Logical  logical_function=AND  inputs=4  precision=Full  arith_type=Unsigned  n_bits=8  bin_pt=2  align_bp=on  latency=0  explicit_period=off  period=1  en=off  dbl_ovrd=off  show_param=off
      settings: xl_area=[0, 0, 0, 0, 0, 0, 0]
  fifo_full : xbsIndex_r3/Logical  logical_function=OR  inputs=4  precision=Full  arith_type=Unsigned  n_bits=8  bin_pt=2  align_bp=on  latency=0  explicit_period=off  period=1  en=off  dbl_ovrd=off  show_param=off
      settings: xl_area=[0, 0, 0, 0, 0, 0, 0]
  fifo_full1 : xbsIndex_r3/Logical  logical_function=OR  inputs=3  precision=Full  arith_type=Unsigned  n_bits=8  bin_pt=2  align_bp=on  latency=0  explicit_period=off  period=1  en=off  dbl_ovrd=off  show_param=off
      settings: xl_area=[0, 0, 0, 0, 0, 0, 0]
  flush : xps_library/software register  Tag=xps:sw_reg  io_dir=From Processor  arith_type=Unsigned  bitwidth=32  bin_pt=0  sample_period=1  gw_name=test_10gbe_mux_pack_mux_pack_it1_flush_user_data_out
  fwft_fifo_data : Subsystem
  fwft_fifo_ip_addr : Subsystem
  in0_data : Subsystem  mask{depth_bits=ceil(log2(max(max_packet_size_0,max_packet_size_1))) +1}
      mask prompts: depth_bits "Fifo Depth (2^?):"
      mask help: A rollback fifo behaves as a normal fifo, except that data which are written in have to be "committed" before they become available for readout. Moreover, any data which are written in and have not been committed can be "discarded", and will never be made available for readout.
  in0_ip_addr : Subsystem  mask{depth_bits=ceil(log2(ceil((max_packet_size_1 / min_packet_size_0))))+1}
      mask prompts: depth_bits "Fifo Depth (2^?):"
      mask help: A rollback fifo behaves as a normal fifo, except that data which are written in have to be "committed" before they become available for readout. Moreover, any data which are written in and have not been committed can be "discarded", and will never be made available for readout.
  in1_data : Subsystem  mask{depth_bits=ceil(log2(max(max_packet_size_0,max_packet_size_1))) +1}
      mask prompts: depth_bits "Fifo Depth (2^?):"
      mask help: A rollback fifo behaves as a normal fifo, except that data which are written in have to be "committed" before they become available for readout. Moreover, any data which are written in and have not been committed can be "discarded", and will never be made available for readout.
  in1_ip_addr : Subsystem  mask{depth_bits=ceil(log2(ceil((max_packet_size_0 / min_packet_size_1))))+1}
      mask prompts: depth_bits "Fifo Depth (2^?):"
      mask help: A rollback fifo behaves as a normal fifo, except that data which are written in have to be "committed" before they become available for readout. Moreover, any data which are written in and have not been committed can be "discarded", and will never be made available for readout.
  mux_buffer_full : Scope  NumInputPorts=6
      settings: TimeRange=1500  YMin=100~0~0~-1~-5~-5  YMax=1400~1~1~1~5~5  SaveName=ScopeData11
  mux_out_debug : Scope  NumInputPorts=4
      settings: YMin=0~0~0~0  YMax=4000~1~3.5e+008~1  SaveName=ScopeData5
  sel_1 : xbsIndex_r3/Inverter  latency=0  explicit_period=off  period=1  en=off  dbl_ovrd=off  show_param=off
      settings: xl_area=[0, 0, 0, 0, 0, 0, 0]
  status : xps_library/software register  Tag=xps:sw_reg  io_dir=To Processor  arith_type=Unsigned  bitwidth=32  bin_pt=0  sample_period=1  gw_name=test_10gbe_mux_pack_mux_pack_it1_status_user_data_in
  we_sel : xbsIndex_r3/Mux  inputs=2  precision=Full  arith_type="Signed  (2's comp)"  n_bits=8  bin_pt=2  quantization=Truncate  overflow=Wrap  latency=0  explicit_period=off  period=1  en=off  dbl_ovrd=off  show_param=off  mux_type=off  use_rpm=off  gen_core=off
      settings: xl_area=[0, 0, 0, 0, 0, 0, 0]
  data : Outport
  valid : Outport  Port=2
  ip_addr : Outport  Port=3
  eof : Outport  Port=4
  discard : Outport  Port=5
  buffer_overflow : Outport  Port=6
  buffer_empty : Outport  Port=7
  ack_0 : Outport  Port=8
  ack_1 : Outport  Port=9
  wires:
  in0_data/2(valid) -> [valid_out0]
  in0_data/1(dout) -> Slice1/1, [d_out0]
  discard_0/1 -> in0_data/4(discard), in0_ip_addr/4(discard)
  in0_data/5(empty) -> [in0_data_empty]
  Concat/1 -> in0_data/1(din)
  Slice1/1 -> [eof0]
  in0_data/4(full) -> Inverter4/1, [in0_data_full]
  Inverter4/1 -> enable_rd_from_2/2
  in0_ip_addr/4(full) -> [in0_ip_full]
  in1_data/1(dout) -> Slice3/1, [d_out1]
  discard_1/1 -> in1_ip_addr/4(discard), in1_data/4(discard)
  in1_data/5(empty) -> [in1_data_empty]
  Concat1/1 -> in1_data/1(din)
  Slice3/1 -> Mux3/2, [eof1]
  in1_data/4(full) -> Inverter5/1, [in1_data_full]
  Inverter5/1 -> enable_rd_from_3/2
  enable_rd_from_2/1 -> in0_ip_addr/3(commit), in0_ip_addr/2(we)
  enable_rd_from_3/1 -> in1_ip_addr/3(commit), in1_ip_addr/2(we)
  in1_ip_addr/4(full) -> [in1_ip_full]
  Register/1 -> [in_sel]
  Constant12/1 -> Register/1
  d_in_0/1 -> Concat/2
  valid_0/1 -> in0_data/2(we)
  dest_ip_0/1 -> in0_ip_addr/1(din)
  eof_0/1 -> enable_rd_from_2/1, in0_data/3(commit), Concat/1
  d_in_1/1 -> Concat1/2
  valid_1/1 -> in1_data/2(we)
  dest_ip_1/1 -> in1_ip_addr/1(din)
  eof_1/1 -> enable_rd_from_3/1, Concat1/1, in1_data/3(commit)
  in0_data/3(wr_ack) -> ack_0/1
  in1_data/3(wr_ack) -> ack_1/1
  Convert2/1 -> valid/1
  0_eof_AND_1_not_empty/1 -> Convert3/1
  1_eof_AND_0_valid/1 -> Convert4/1
  Convert3/1 -> Register/3
  Convert4/1 -> Register/2
  Constant13/1 -> discard/1
  Slice2/1 -> eof/1, enable_rd_from_1/2
  dout_and_eof_sel/1 -> Slice5/1, fwft_fifo_data/1(din), Slice7/1, Slice6/1
  Slice4/1 -> data/1
  fwft_fifo_data/2(valid) -> Convert2/1
  we_sel/1 -> fwft_fifo_data/2(we), Gateway Out9/1
  rd_ack/1 -> enable_rd_from_1/1, Mux4/2
  dest_ip_sel/1 -> Gateway Out10/1, fwft_fifo_ip_addr/1(din)
  Slice5/1 -> fwft_fifo_ip_addr/2(we)
  fwft_fifo_ip_addr/1(dout) -> ip_addr/1
  Gateway Out12/1 -> mux_out_debug/1
  Gateway Out9/1 -> mux_out_debug/2
  Gateway Out10/1 -> mux_out_debug/3
  Gateway Out11/1 -> mux_out_debug/4
  fwft_fifo_data/1(dout) -> Slice4/1, Slice2/1
  fifo_full1/1 -> buffer_overflow/1
  fwft_fifo_data/3(overflow) -> fifo_full1/1, Gateway Out19/1
  fwft_fifo_ip_addr/3(overflow) -> fifo_full1/2, Gateway Out20/1
  fifo_full/1 -> fifo_full1/3
  fifo_empty/1 -> buffer_empty/1
  Slice7/1 -> Gateway Out11/1
  Gateway Out17/1 -> mux_buffer_full/1
  Gateway Out18/1 -> mux_buffer_full/2
  Gateway Out15/1 -> mux_buffer_full/3
  Gateway Out16/1 -> mux_buffer_full/4
  Gateway Out19/1 -> mux_buffer_full/5
  Gateway Out20/1 -> mux_buffer_full/6
  Constant/1 -> flush/1
  flush/1 -> Slice/1
  Mux/1 -> in0_data/5(rd_ack)
  Constant1/1 -> Mux/3
  Constant2/1 -> Mux1/3
  Mux1/1 -> in0_ip_addr/5(rd_ack)
  Constant3/1 -> Mux2/3
  Mux2/1 -> in1_data/5(rd_ack)
  Constant4/1 -> Mux3/3
  Mux3/1 -> in1_ip_addr/5(rd_ack)
  [flush_buffers] -> Mux/1
  [flush_buffers] -> Mux1/1
  [flush_buffers] -> Mux2/1
  [flush_buffers] -> Mux3/1
  Constant5/1 -> Mux4/3
  [flush_buffers] -> Mux4/1
  Mux4/1 -> fwft_fifo_data/3(ack)
  Constant6/1 -> Mux5/3
  [flush_buffers] -> Mux5/1
  Mux5/1 -> fwft_fifo_ip_addr/3(ack)
  enable_rd_from_1/1 -> Mux5/2
  Slice/1 -> [flush_buffers]
  Inverter/1 -> 0_eof_AND_1_not_empty/2
  Inverter1/1 -> 1_eof_AND_0_valid/1
  [in0_ip_empty] -> fifo_empty/1
  [in0_data_empty] -> fifo_empty/2
  in0_ip_addr/5(empty) -> [in0_ip_empty]
  [in0_ip_full] -> fifo_full/1
  [in0_data_full] -> fifo_full/2
  [in1_ip_full] -> fifo_full/3
  [in1_data_full] -> fifo_full/4
  [in1_ip_empty] -> fifo_empty/3
  [in1_data_empty] -> fifo_empty/4
  in1_ip_addr/5(empty) -> [in1_ip_empty]
  [in1_ip_full] -> Gateway Out15/1
  [in1_data_full] -> Gateway Out16/1
  [in0_ip_full] -> Gateway Out17/1
  [in0_data_full] -> Gateway Out18/1
  [in1_data_empty] -> Inverter/1
  [in0_data_empty] -> Inverter1/1
  [eof0] -> 0_eof_AND_1_not_empty/1
  [eof0] -> Mux1/2
  [eof1] -> 1_eof_AND_0_valid/2
  [in_sel] -> dout_and_eof_sel/1
  [in_sel] -> sel_1/1
  sel_1/1 -> Mux/2
  [in_sel] -> Mux2/2
  Slice6/1 -> Gateway Out12/1
  [d_out0] -> dout_and_eof_sel/2
  [valid_out0] -> we_sel/2
  [valid_out1] -> we_sel/3
  in0_ip_addr/1(dout) -> [ip_out0]
  [ip_out0] -> dest_ip_sel/2
  [ip_out1] -> dest_ip_sel/3
  in1_data/2(valid) -> [valid_out1]
  in1_ip_addr/1(dout) -> [ip_out1]
  [d_out1] -> dout_and_eof_sel/3
  [in_sel] -> dest_ip_sel/1
  [in_sel] -> we_sel/1
  Constant7/1 -> Concat2/1
  [in0_ip_full] -> Convert1/1
  [in0_data_full] -> Convert5/1
  [in1_ip_full] -> Convert6/1
  [in1_data_full] -> Convert7/1
  [in0_ip_empty] -> Convert8/1
  [in0_data_empty] -> Convert9/1
  [in1_ip_empty] -> Convert10/1
  [in1_data_empty] -> Convert11/1
  Concat2/1 -> status/1
  [in_sel] -> Convert12/1
  Convert1/1 -> Concat2/2
  Convert5/1 -> Concat2/3
  Convert6/1 -> Concat2/4
  Convert7/1 -> Concat2/5
  Convert8/1 -> Concat2/6
  Convert10/1 -> Concat2/8
  Convert9/1 -> Concat2/7
  Convert11/1 -> Concat2/9
  Convert12/1 -> Concat2/10
